simulink model "State_space"  (R2019a)
settings: Solver=ode1  StartTime=0.0  StopTime=50  FixedStep=0.01  RelTol=1e-3
settings Model: Creator=ADMIN  LastModifiedBy=ADMIN
settings SolverCC: AlgebraicLoopSolver=LineSearch

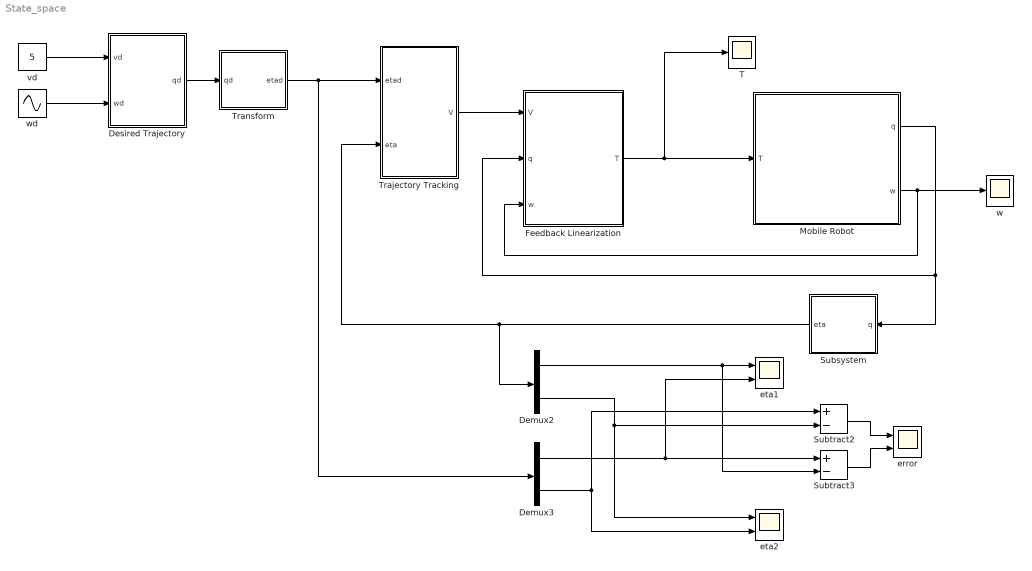
== system State_space ==
  Demux2 : Demux  Outputs=2
  Demux3 : Demux  Outputs=2
  Desired Trajectory : Subsystem  mask{xd0=0.707, yd0=0.707, thetad0=0}
      mask TypeOptions xd0: xd0/InitialCondition
      mask TypeOptions yd0: yd0/InitialCondition
      mask TypeOptions thetad0: thetad0/InitialCondition
  Feedback Linearization : Subsystem
  Mobile Robot : Subsystem  mask{x0=3, y0=7, theta0=-pi, wr0=2, wl0=3}
      mask TypeOptions x0: x0/InitialCondition
      mask TypeOptions y0: y0/InitialCondition
      mask TypeOptions theta0: theta0/InitialCondition
      mask TypeOptions wr0: wr0/InitialCondition
      mask TypeOptions wl0: wl0/InitialCondition
  Subsystem : Subsystem
  Subtract2 : Sum  Inputs=+-
  Subtract3 : Sum  Inputs=+-
  T : Scope
  Trajectory Tracking : Subsystem  mask{Kd=[10;20], Kp=[30;60]}
      mask TypeOptions Kd: KD1/Gain
      mask TypeOptions Kp: KP1/Gain
  Transform : Subsystem
  error : Scope  NumInputPorts=2
  eta1 : Scope  NumInputPorts=2
  eta2 : Scope  NumInputPorts=2
  vd : Constant  Value=5
  w : Scope
  wd : Sin  Amplitude=3  Frequency=0.4*pi  SampleTime=0
  wires:
  Feedback Linearization/1(T) -> T/1, Mobile Robot/1(T)
  Trajectory Tracking/1(V) -> Feedback Linearization/1(V)
  vd/1 -> Desired Trajectory/1(vd)
  wd/1 -> Desired Trajectory/2(wd)
  Mobile Robot/2(w) -> w/1, Feedback Linearization/3(w)
  Mobile Robot/1(q) -> Subsystem/1(q), Feedback Linearization/2(q)
  Desired Trajectory/1(qd) -> Transform/1(qd)
  Demux2/2 -> Subtract2/2, eta2/1
  Demux3/2 -> Subtract2/1, eta2/2
  Subsystem/1(eta) -> Demux2/1, Trajectory Tracking/2(eta)
  Transform/1(etad) -> Demux3/1, Trajectory Tracking/1(etad)
  Subtract2/1 -> error/1
  Demux2/1 -> Subtract3/2, eta1/1
  Demux3/1 -> eta1/2, Subtract3/1
  Subtract3/1 -> error/2

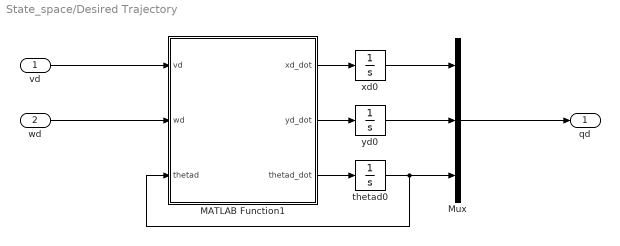
== system State_space/Desired Trajectory ==
  vd : Inport
  wd : Inport  Port=2
  MATLAB Function1 : MATLAB Function  TreatAsAtomicUnit=on
  Mux : Mux  Inputs=3
  thetad0 : Integrator  InitialCondition=thetad0
  xd0 : Integrator  InitialCondition=xd0
  yd0 : Integrator  InitialCondition=yd0
  qd : Outport
  wires:
  wd/1 -> MATLAB Function1/2(wd)
  vd/1 -> MATLAB Function1/1(vd)
  MATLAB Function1/1(xd_dot) -> xd0/1
  MATLAB Function1/2(yd_dot) -> yd0/1
  MATLAB Function1/3(thetad_dot) -> thetad0/1
  thetad0/1 -> Mux/3, MATLAB Function1/3(thetad)
  xd0/1 -> Mux/1
  yd0/1 -> Mux/2
  Mux/1 -> qd/1

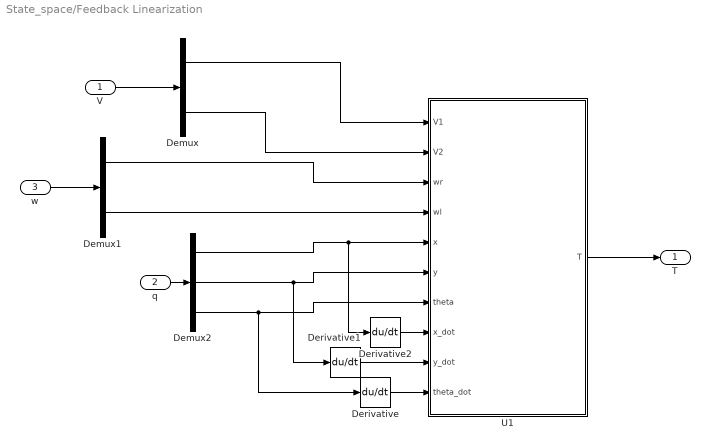
== system State_space/Feedback Linearization ==
  V : Inport
  q : Inport  Port=2
  w : Inport  Port=3
  Demux : Demux  Outputs=2
  Demux1 : Demux  Outputs=2
  Demux2 : Demux  Outputs=3
  Derivative : Derivative
  Derivative1 : Derivative
  Derivative2 : Derivative
  U1 : MATLAB Function  TreatAsAtomicUnit=on
  T : Outport
  wires:
  V/1 -> Demux/1
  Demux/1 -> U1/1(V1)
  Demux/2 -> U1/2(V2)
  U1/1(T) -> T/1
  w/1 -> Demux1/1
  Derivative/1 -> U1/10(theta_dot)
  Demux1/1 -> U1/3(wr)
  Demux1/2 -> U1/4(wl)
  q/1 -> Demux2/1
  Demux2/1 -> Derivative2/1, U1/5(x)
  Demux2/2 -> Derivative1/1, U1/6(y)
  Demux2/3 -> Derivative/1, U1/7(theta)
  Derivative1/1 -> U1/9(y_dot)
  Derivative2/1 -> U1/8(x_dot)

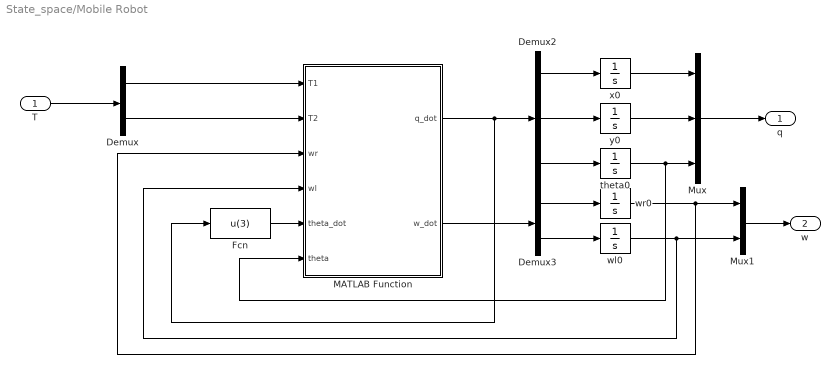
== system State_space/Mobile Robot ==
  T : Inport
  Demux : Demux  Outputs=2
  Demux2 : Demux  Outputs=3
  Demux3 : Demux  Outputs=2
  Fcn : Fcn  Expr=u(3)
  MATLAB Function : MATLAB Function  TreatAsAtomicUnit=on
  Mux : Mux  Inputs=3
  Mux1 : Mux  Inputs=2
  theta0 : Integrator  InitialCondition=theta0
  wl0 : Integrator  InitialCondition=wl0
  wr0 : Integrator  InitialCondition=wr0
  x0 : Integrator  InitialCondition=x0
  y0 : Integrator  InitialCondition=y0
  q : Outport
  w : Outport  Port=2
  wires:
  T/1 -> Demux/1
  Demux/1 -> MATLAB Function/1(T1)
  Demux/2 -> MATLAB Function/2(T2)
  Demux2/1 -> x0/1
  Demux2/2 -> y0/1
  Demux2/3 -> theta0/1
  theta0/1 -> MATLAB Function/6(theta), Mux/3
  y0/1 -> Mux/2
  x0/1 -> Mux/1
  Mux/1 -> q/1
  MATLAB Function/1(q_dot) -> Fcn/1, Demux2/1
  Mux1/1 -> w/1
  MATLAB Function/2(w_dot) -> Demux3/1
  Demux3/1 -> wr0/1
  Demux3/2 -> wl0/1
  wr0/1 -> MATLAB Function/3(wr), Mux1/1
  wl0/1 -> MATLAB Function/4(wl), Mux1/2
  Fcn/1 -> MATLAB Function/5(theta_dot)

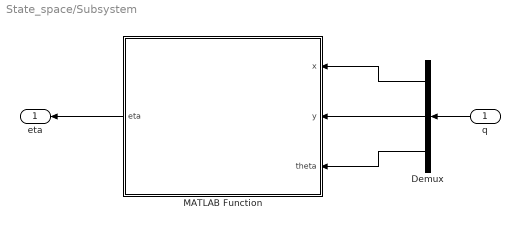
== system State_space/Subsystem ==
  q : Inport
  Demux : Demux  Outputs=3
  MATLAB Function : MATLAB Function  TreatAsAtomicUnit=on
  eta : Outport
  wires:
  MATLAB Function/1(eta) -> eta/1
  q/1 -> Demux/1
  Demux/2 -> MATLAB Function/2(y)
  Demux/1 -> MATLAB Function/1(x)
  Demux/3 -> MATLAB Function/3(theta)

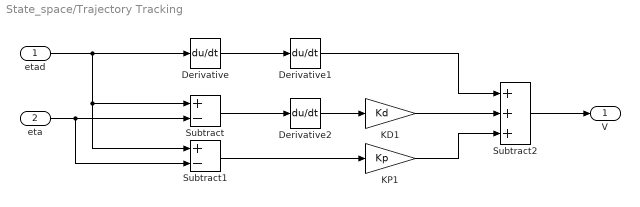
== system State_space/Trajectory Tracking ==
  etad : Inport
  eta : Inport  Port=2
  Derivative : Derivative
  Derivative1 : Derivative
  Derivative2 : Derivative
  KD1 : Gain  Gain=Kd
  KP1 : Gain  Gain=Kp
  Subtract : Sum  Inputs=+-
  Subtract1 : Sum  Inputs=+-
  Subtract2 : Sum  Inputs=+++
  V : Outport
  wires:
  Derivative/1 -> Derivative1/1
  Subtract/1 -> Derivative2/1
  Subtract1/1 -> KP1/1
  Derivative1/1 -> Subtract2/1
  KP1/1 -> Subtract2/3
  eta/1 -> Subtract1/2, Subtract/2
  etad/1 -> Subtract1/1, Subtract/1, Derivative/1
  Derivative2/1 -> KD1/1
  KD1/1 -> Subtract2/2
  Subtract2/1 -> V/1

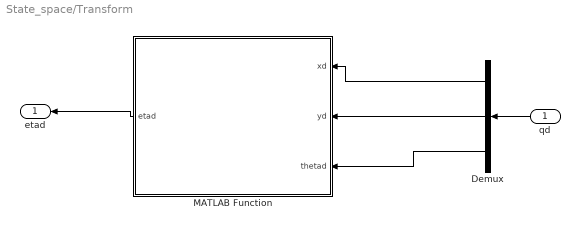
== system State_space/Transform ==
  qd : Inport
  Demux : Demux  Outputs=3
  MATLAB Function : MATLAB Function  TreatAsAtomicUnit=on
  etad : Outport
  wires:
  MATLAB Function/1(etad) -> etad/1
  qd/1 -> Demux/1
  Demux/1 -> MATLAB Function/1(xd)
  Demux/2 -> MATLAB Function/2(yd)
  Demux/3 -> MATLAB Function/3(thetad)

== matlab function State_space/Feedback Linearization/U1 ==
  data: V1 input; V2 input; wr input; wl input; x input; y input; theta input; x_dot input; y_dot input; theta_dot input; T output
function T = fcn(V1, V2, wr, wl, x, y, theta, x_dot, y_dot, theta_dot)
%% Parameters
r = 0.05;    %% (m) Radius of wheels
L = 0.27/2;  %% (m) 2L: Distance between two driving wheels
m = 4 ;      %% (kg) Mass of robot
I = 2.5;     %% (kg.m^2) Moment of inertia of whole robot
d = 0.05;    %% (m) Distance from point p0 to point pc
a = r/2;
b = r/(2*L);
%%
w = [wr; wl];
V = [V1; V2];       
Phi = [b, -b;
       2*a*(x*cos(theta)+y*sin(theta)),   2*a*(x*cos(theta)+y*sin(theta))];
Phi_dot = [0,   0;
           2*a*(cos(theta)*(x_dot+y*theta_dot)+sin(theta)*(-x*theta_dot+y_dot)),2*a*(cos(theta)*(x_dot+y*theta_dot)+sin(theta)*(-x*theta_dot+y_dot))];
M_ = [m*a^2 + I*b^2,    m*a^2 - I*b^2;
      m*a^2 - I*b^2,    m*a^2 + I*b^2];
C_ = [0,        -2*a*b*d*theta_dot;
      2*a*b*d*theta_dot,    0]; 
B_ = [1,  0;  0,  1];
%%
Alpha = Phi_dot*w - Phi*inv(M_)*C_*w;
Beta = Phi*inv(M_)*B_;
%%
T = inv(Beta)*( - Alpha + V );
end
%%

== matlab function State_space/Mobile Robot/MATLAB Function ==
  data: T1 input; T2 input; wr input; wl input; theta_dot input; theta input; q_dot output; w_dot output
function [q_dot, w_dot] = fcn(T1, T2, wr, wl, theta_dot, theta)
%% Parameters
r = 0.05;    %% (m) Radius of wheels
L = 0.27/2;  %% (m) 2L: Distance between two driving wheels
m = 4 ;      %% (kg) Mass of robot
I = 2.5;     %% (kg.m^2) Moment of inertia of whole robot
d = 0.05;    %% (m) Distance from point p0 to point pc
a = r/2;
b = r/(2*L);
%% M*q_2dot + C*q_dot = B*T
Sk = [a*cos(theta), a*cos(theta);
      a*sin(theta), a*sin(theta);
            b,          -b];
M_ = [m*a^2 + I*b^2,    m*a^2 - I*b^2;
      m*a^2 - I*b^2,    m*a^2 + I*b^2];

C_ = [0,        -2*a*b*d*theta_dot;
      2*a*b*d*theta_dot,    0]; 

B_ = [1,  0;  0,  1];

w = [wr ; wl];
T = [T1 ; T2];
%%  q_dot, W_dot
    q_dot = Sk*w;
    w_dot = inv(M_)*( -C_*w + B_*T);
end
%%

== matlab function State_space/Subsystem/MATLAB Function ==
  data: x input; eta output; y input; theta input
function eta = fcn(x, y,theta)
eta = [theta;
       x^2 + y^2];
end

== matlab function State_space/Transform/MATLAB Function ==
  data: xd input; etad output; yd input; thetad input
function etad = fcn(xd, yd, thetad)
etad = [thetad;
       xd^2 + yd^2];
end

== matlab function State_space/Desired Trajectory/MATLAB Function1 ==
  data: vd input; xd_dot output; wd input; yd_dot output; thetad_dot output; thetad input
function [xd_dot, yd_dot, thetad_dot] = fcn(vd, wd, thetad)
xd_dot = vd*cos(thetad);
yd_dot = vd*sin(thetad);
thetad_dot = wd;

end
